simulink model "Chart11"  (R2022b)
settings: Solver=FixedStepDiscrete  StartTime=0.0  StopTime=1  FixedStep=0.01  RelTol=1e-3  EnableMultiTasking=on
settings Model: Creator=ahmed  LastModifiedBy=Mohamed
settings SolverCC: PositivePriorityOrder=on
settings DataIOCC: SaveOutput=off  SaveTime=off
settings OptimizationCC: EnhancedBackFolding=on  PassReuseOutputArgsAs=Individual arguments  ZeroExternalMemoryAtStartup=off  ZeroInternalMemoryAtStartup=off  MaxStackSize=64  OptimizeBlockOrder=speed  DifferentSizesBufferReuse=on  OptimizationCustomize=off  EfficientTunableParamExpr=on
settings DebuggingCC: ParameterTunabilityLossMsg=error
settings HardwareCC: ProdBitPerPointer=32  ProdBitPerSizeT=32  ProdBitPerPtrDiffT=32  ProdLargestAtomicInteger=Long  ProdLargestAtomicFloat=Double  ProdWordSize=32  ProdLongLongMode=on  ProdHWDeviceType=ARM Compatible->ARM Cortex
settings ModelReferenceCC: PropagateVarSize=During execution
settings RTWCC: Description=Embedded Coder  SystemTargetFile=ert.tlc  HardwareBoard=Raspberry Pi  TLCOptions="-aInlineSetEventsForThisBaseRateFcn=TLC_FALSE -aSuppressMultiTaskScheduler=TLC_FALSE  -aRateBasedStepFcn=0"  TemplateMakefile=ert_default_tmf  Toolchain=GNU GCC Embedded Linux  BuildConfiguration=Faster Runs
settings CodeAppCC: ForceParamTrailComments=on  IgnoreCustomStorageClasses=off  OperatorAnnotations=on  SimulinkDataObjDesc=on  SFDataObjDesc=on  InsertBlockDesc=on
settings ERTTargetCC: SupportContinuousTime=on  SupportVariableSizeSignals=on  ExtModeTransport=2  ExtModeStaticAlloc=on  ExtModeMexFile=ext_xcp  ExtModeIntrfLevel=Level2 - Open

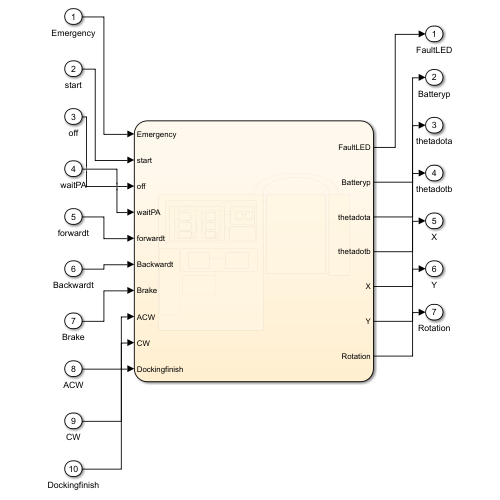
[thumbnail: Simulink's stored preview of the top-level diagram]
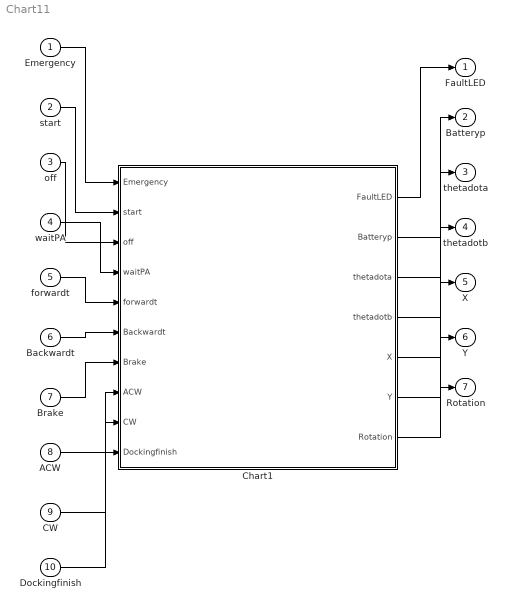
== system Chart11 ==
  Emergency : Inport  OutDataTypeStr=double  PortDimensions=1
  start : Inport  Port=2  OutDataTypeStr=double  PortDimensions=1
  off : Inport  Port=3  OutDataTypeStr=double  PortDimensions=1
  waitPA : Inport  Port=4  OutDataTypeStr=double  PortDimensions=1
  forwardt : Inport  Port=5  OutDataTypeStr=double  PortDimensions=1
  Backwardt : Inport  Port=6  OutDataTypeStr=double  PortDimensions=1
  Brake : Inport  Port=7  OutDataTypeStr=double  PortDimensions=1
  ACW : Inport  Port=8  OutDataTypeStr=double  PortDimensions=1
  CW : Inport  Port=9  OutDataTypeStr=double  PortDimensions=1
  Dockingfinish : Inport  Port=10  OutDataTypeStr=double  PortDimensions=1
  Chart1 : Stateflow chart  TreatAsAtomicUnit=on
  FaultLED : Outport  OutDataTypeStr=double  PortDimensions=1  SampleTime=[0.01,0]
  Batteryp : Outport  Port=2  OutDataTypeStr=double  PortDimensions=1  SampleTime=[0.01,0]
  thetadota : Outport  Port=3  OutDataTypeStr=double  PortDimensions=1  SampleTime=[0.01,0]
  thetadotb : Outport  Port=4  OutDataTypeStr=double  PortDimensions=1  SampleTime=[0.01,0]
  X : Outport  Port=5  OutDataTypeStr=double  PortDimensions=1  SampleTime=[0.01,0]
  Y : Outport  Port=6  OutDataTypeStr=double  PortDimensions=1  SampleTime=[0.01,0]
  Rotation : Outport  Port=7  OutDataTypeStr=double  PortDimensions=1  SampleTime=[0.01,0]
  wires:
  Emergency/1 -> Chart1/1(Emergency)
  start/1 -> Chart1/2(start)
  off/1 -> Chart1/3(off)
  waitPA/1 -> Chart1/4(waitPA)
  forwardt/1 -> Chart1/5(forwardt)
  Backwardt/1 -> Chart1/6(Backwardt)
  Brake/1 -> Chart1/7(Brake)
  ACW/1 -> Chart1/8(ACW)
  CW/1 -> Chart1/9(CW)
  Dockingfinish/1 -> Chart1/10(Dockingfinish)
  Chart1/1(FaultLED) -> FaultLED/1
  Chart1/2(Batteryp) -> Batteryp/1
  Chart1/3(thetadota) -> thetadota/1
  Chart1/4(thetadotb) -> thetadotb/1
  Chart1/5(X) -> X/1
  Chart1/6(Y) -> Y/1
  Chart1/7(Rotation) -> Rotation/1

== stateflow chart Chart11/Chart1 ==
  state ON
    state Active_task [parallel]
      settings: executionOrder=1
      state Motion
        state Translational [parallel]
          exit:
          t=0;
          settings: executionOrder=1
          state Forward
            entry:
            t=1
          state Backward
            entry:
            t=-1
          state none
            entry:
            t=0
          ON.Active_task.Motion.Translational.none -> Forward [order 2] : [forwardt==1]
          Forward -> ON.Active_task.Motion.Translational.none [order 1] : [Brake==1]
          Forward -> Backward [order 2] : [Backwardt==1]
          Backward -> Forward [order 1] : [forwardt==1]
          ON.Active_task.Motion.Translational.none -> Backward [order 1] : [Backwardt==1]
          Backward -> ON.Active_task.Motion.Translational.none [order 2] : [Brake==1]
          (default) -> ON.Active_task.Motion.Translational.none
          ON.Active_task.Motion.Translational.none -> ON.Active_task.Motion.Translational.none [order 3] : [Brake==1]
        state Rotational [parallel]
          exit:
          r=0;
          settings: executionOrder=2
          state CLCK_WISE
            entry:
            r=-1
          state Anti_CLCKWISE
            entry:
            r=1
          state none
            entry:
            r=0
          ON.Active_task.Motion.Rotational.none -> CLCK_WISE [order 2] : [CW==1]
          CLCK_WISE -> ON.Active_task.Motion.Rotational.none [order 2] : [Brake==1]
          Anti_CLCKWISE -> CLCK_WISE [order 2] : [CW==1]
          CLCK_WISE -> Anti_CLCKWISE [order 1] : [ACW==1]
          ON.Active_task.Motion.Rotational.none -> Anti_CLCKWISE [order 1] : [ACW==1]
          Anti_CLCKWISE -> ON.Active_task.Motion.Rotational.none [order 1] : [Brake==1]
          (default) -> ON.Active_task.Motion.Rotational.none
          ON.Active_task.Motion.Rotational.none -> ON.Active_task.Motion.Rotational.none [order 3] : [Brake==1]
      state Charging_station
        state Docking
          exit:
          d=1;
        state Docked
          exit:
          d=0;
        Docking -> Docked : [Dockingfinish==1]
        (default) -> Docking
      state Waiting
        entry:
        r=0;
        t=0;
        during:
        if ( forwardt || Backwardt || CW || ACW == 1)
        g=1;
        end
        exit:
        g=0;
      Motion -> Charging_station [order 2] : [Batteryp<=30]
      (default) -> Motion
      Charging_station -> Motion : [Batteryp==100]
      Waiting -> Motion : [g==1 & waitPA ==0]
      Motion -> Waiting [order 1] : [waitPA==1]
    state Continuous [parallel]
      entry:
      %setting DCmotor Conditions
      J=0.01;
      b=0.1;
      Ke=0.01;
      Kt=0.01;
      R=1;
      L=0.5;
      Ts = 0.01;
      %%setting AGV parameters
      radius = 1;
      wheelradius=0.1;
      during:
      %using t and r to find motor speeds
      Va_Desired = 5*(t + (0.4/2)* r);
      Vb_Desired=  5*(t - (0.4/2)* r);
      %First Motor Equations
      thetadoubledota = (1/J)*(Kt*ia-b*thetadota);
      idota = (1/L)*(-R*ia+input_MotorA-Ke*thetadota);
      ia=ia+idota*Ts;
      thetadota=thetadota+thetadoubledota*Ts;
      %%second Motor Equations
      thetadoubledotb = (1/J)*(Kt*ib-b*thetadotb);
      idotb = (1/L)*(-1*ib+input_MotorB-Ke*thetadotb);
      ib=ib+idotb*Ts;
      thetadotb=thetadotb+thetadoubledotb*Ts;
      %%updating Current taken from battery
      Id=ia+ib;
      %% Updating X Y and Rotation of AGV
      Va =  thetadota* wheelradius;
      Vb = thetadotb*wheelradius;
      Vt=(Va+Vb)/2;
      rotationSpeed=(Va-Vb)/radius;
      Rotation = Rotation+rotationSpeed*Ts;
      X=X+Vt*cos(Rotation)*Ts;
      Y=Y+Vt*sin(Rotation)*Ts;
      settings: executionOrder=3
    state Battery_management [parallel]
      settings: executionOrder=2
      state Charging
        during:
        SOC = SOC + I*Ts
        if(SOC>=100000)
        SOC=100000
        end
        Batteryp = (SOC/100000)*100
      state Discharging
        during:
        SOC = SOC - abs(Id)*Ts
        if(SOC>=100000)
        SOC=100000
        end
        Batteryp = (SOC/100000)*100
      (default) -> Discharging
      Charging -> Discharging : [d==0]
      Discharging -> Charging : [d==1]
    state PID_Controller [parallel]
      %% First Controller
      Kp=40;
      Ki=100;
      Kd=0.01;
      Error_old_MotorA= Error_MotorA;
      Error_MotorA =Va_Desired/wheelradius-thetadota;
      inte_MotorA = inte_MotorA+Error_MotorA*Ts;
      Diff_MotorA = (Error_MotorA-Error_old_MotorA)/Ts;
      input_MotorA = Kp*Error_MotorA+Ki*inte_MotorA+Kd*Diff_MotorA;
      %% Second Controller
      Kp=40;
      Ki=100;
      Kd=0.01;
      Error_old_MotorB= Error_MotorB;
      Error_MotorB =Vb_Desired/wheelradius-thetadotb;
      inte_MotorB = inte_MotorB+Error_MotorB*Ts;
      Diff_MotorB = (Error_MotorB-Error_old_MotorB)/Ts;
      input_MotorB = Kp*Error_MotorB+Ki*inte_MotorB+Kd*Diff_MotorB;
      settings: executionOrder=4
  state OFF
    entry:
    r=0
    t=0
    thetadota=0;
    thetadotb=0;
  state Emergency
    entry:
    FaultLED=1;
    r=0;
    t=0;
    thetadota=0;
    thetadotb=0;
    exit:
    FaultLED=0;
  Emergency -> ON : [start==1 && Emergency==0]
  ON -> Emergency [order 2] : [Emergency==1]
  (default) -> OFF
  OFF -> ON : [start==1]
  ON -> OFF [order 1] : [off==1]
  data: FaultLED output; Emergency input; start input; off input; waitPA input; forwardt input; Backwardt input; Brake input; ACW input; CW input; Batteryp output =100; I local =100; SOC local =100000; d local =0; Dockingfinish input; g local =0; t local; r local; Id local =0; J local =0; Ke local =0; Kt local =0; L local =0; R local =0; Ts local =0; Va local =0; Vb local =0; b local =0; ia local =0; ib local =0; idota local =0; idotb local =0; thetadoubledota local =0; thetadoubledotb local =0; thetadota output =0; thetadotb output =0; Diff_MotorA local =0; Diff_MotorB local =0; Error_MotorA local =0; Error_MotorB local =0; Error_old_MotorA local =0; Error_old_MotorB local =0; Kd local =0; Ki local =00; Kp local =00; input_MotorA local =0; input_MotorB local =0; inte_MotorA local =0; inte_MotorB local =0; radius local =0; Va_Desired local =0; Vb_Desired local =0; Vt local =0; rotationSpeed local =0; wheelradius local =0; X output =0; Y output =0; Rotation output =0
